simulink model "silnik_sprz_stan"  (R2025b)
settings: Solver=ode3  StartTime=0.0  StopTime=tend  FixedStep=0.001  RelTol=1e-3  EnableMultiTasking=on
undefined symbols (not defined in the file): K, kstat, tend
settings Model: Creator=Jacek  LastModifiedBy=janek
settings SolverCC: AlgebraicLoopSolver=TrustRegion
settings DataIOCC: LimitDataPoints=on  SaveFormat=Array  ReturnWorkspaceOutputs=off
settings OptimizationCC: LifeSpan=inf
settings DebuggingCC: SolverPrmCheckMsg=warning  UnconnectedInputMsg=warning  UnconnectedOutputMsg=warning  UnconnectedLineMsg=warning  SFUnexpectedBacktrackingDiag=warning  SFNoUnconditionalDefaultTransitionDiag=warning  SFExecutionAtInitializationDiag=none  ArithmeticOperatorsInVariantConditions=warning
settings HardwareCC: ProdBitPerPointer=32.0  ProdBitPerSizeT=32.0  ProdBitPerPtrDiffT=32.0  ProdLargestAtomicFloat=None  ProdIntDivRoundTo=Undefined  ProdEndianess=Unspecified  ProdWordSize=32.0  ProdHWDeviceType=32-bit Generic
settings ModelReferenceCC: EnableRefExpFcnMdlSchedulingChecks=on  PropagateSignalLabelsOutOfModel=off
settings SFSimCC: SimUseLocalCustomCode=off  CustomCodeUndefinedFunction=UseInterfaceOnly
settings RTWCC: RTWUseLocalCustomCode=off  GPUComputeCapability=3.5
settings CodeAppCC: StateflowObjectComments=on
settings GRTTargetCC: TargetLangStandard=C89/C90 (ANSI)
settings ConfigComp: CovMetricSettings=dw  CovSaveCumulativeToWorkspaceVar=on  CovSaveSingleToWorkspaceVar=on  CovExternalEMLEnable=off  CovSFcnEnable=off

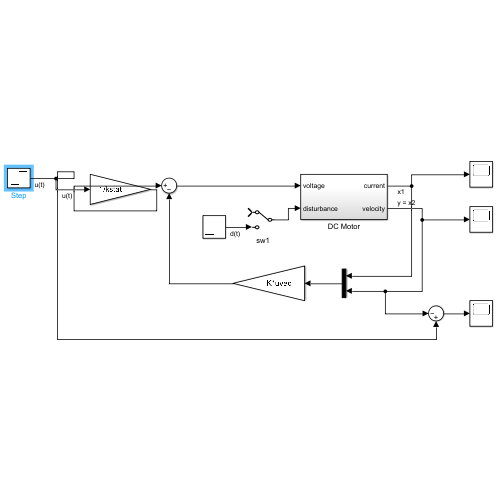
[thumbnail: Simulink's stored preview of the top-level diagram]
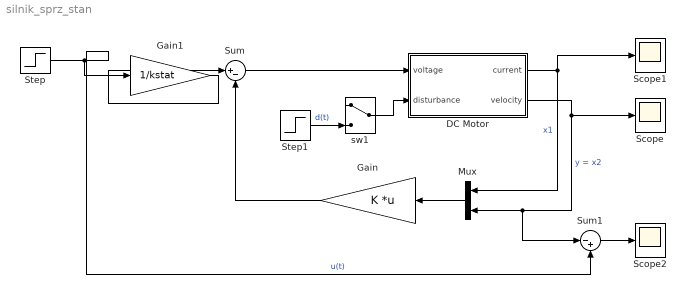
== system silnik_sprz_stan ==
  DC Motor : Subsystem
  Gain : Gain  Gain=K  Multiplication=Matrix(K*u) (u vector)
  Gain1 : Gain  Gain=1/kstat
  Mux : Mux  Inputs=2
  Scope : Scope
      settings: ActiveDisplayYMinimum=9.3466834553198552  ActiveDisplayYMaximum=315.87984890212135
  Scope1 : Scope
      settings: ActiveDisplayYMinimum=-25.502807712796564  ActiveDisplayYMaximum=228.45364208015326
  Scope2 : Scope
      settings: ActiveDisplayYMinimum=-15.87984890212136  ActiveDisplayYMaximum=290.65331654468014  DataLoggingVariableName=ScopeData2
  Step : Step  Time=0  After=300  SampleTime=0
  Step1 : Step  Time=tend/2  After=50  SampleTime=0
  Sum : Sum  Inputs=|+-
  Sum1 : Sum  Inputs=|-+
  sw1 : ManualSwitch
  wires:
  DC Motor/2(velocity) -> Sum1/1, Mux/2, Scope/1  "y = x2"
  Step/1 -> Sum1/2, Gain1/1  "u(t)"
  sw1/1 -> DC Motor/2(disturbance)
  Step1/1 -> sw1/2  "d(t)"
  DC Motor/1(current) -> Mux/1, Scope1/1  "x1"
  Mux/1 -> Gain/1
  Sum/1 -> DC Motor/1(voltage)
  Gain/1 -> Sum/2
  Sum1/1 -> Scope2/1
  Gain1/1 -> Sum/1

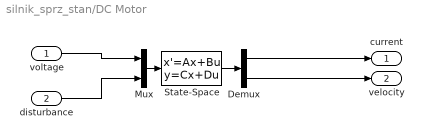
== system silnik_sprz_stan/DC Motor ==
  voltage : Inport
  disturbance : Inport  Port=2
  Demux : Demux  Outputs=2
  Mux : Mux  Inputs=2
  State-Space : StateSpace  A=[-3/0.05, -2.23/0.05; 2.23/0.11, 0]  B=[1/0.05 0; 0 -1/0.11]  C=[1 0;0 1]  D=[0 0; 0 0]  InitialCondition=[0 ;40]
  current : Outport  VectorParamsAs1DForOutWhenUnconnected=off
  velocity : Outport  Port=2  VectorParamsAs1DForOutWhenUnconnected=off
  wires:
  Mux/1 -> State-Space/1
  voltage/1 -> Mux/1
  disturbance/1 -> Mux/2
  State-Space/1 -> Demux/1
  Demux/2 -> velocity/1
  Demux/1 -> current/1
